simulink model "TestAccel"  (R2016a)
settings: Solver=FixedStepAuto  StartTime=0.0  StopTime=inf  FixedStep=1  RelTol=1e-3
libraries: arduinolib x1, EEE481Arduino x1
settings Model: ExtModeTrigDuration=2  Creator=rsjoshi1  LastModifiedBy=rsjoshi1
settings OptimizationCC: OptimizeModelRefInitCode=on  LifeSpan=1  MaxStackSize=64
settings HardwareCC: ProdBitPerPointer=32  ProdLargestAtomicInteger=Long  ProdLargestAtomicFloat=Double  ProdWordSize=32  ProdHWDeviceType=ARM Compatible->ARM Cortex
settings RTWCC: SystemTargetFile=ert.tlc  HardwareBoard=Arduino Due  TemplateMakefile=ert_default_tmf  GenerateReport=on  Toolchain=Arduino ARM v1.6.1  BuildConfiguration=Faster Runs  IncludeHyperlinkInReport=on  LaunchReport=on  GenerateTraceInfo=on  GenerateTraceReport=on  GenerateTraceReportSl=on  GenerateTraceReportSf=on  GenerateTraceReportEml=on
settings CodeAppCC: ForceParamTrailComments=on  IgnoreCustomStorageClasses=off  OperatorAnnotations=on  SimulinkDataObjDesc=on  SFDataObjDesc=on  MATLABFcnDesc=on  InsertBlockDesc=on  MATLABSourceComments=on
settings ERTTargetCC: SupportContinuousTime=on  SupportVariableSizeSignals=on

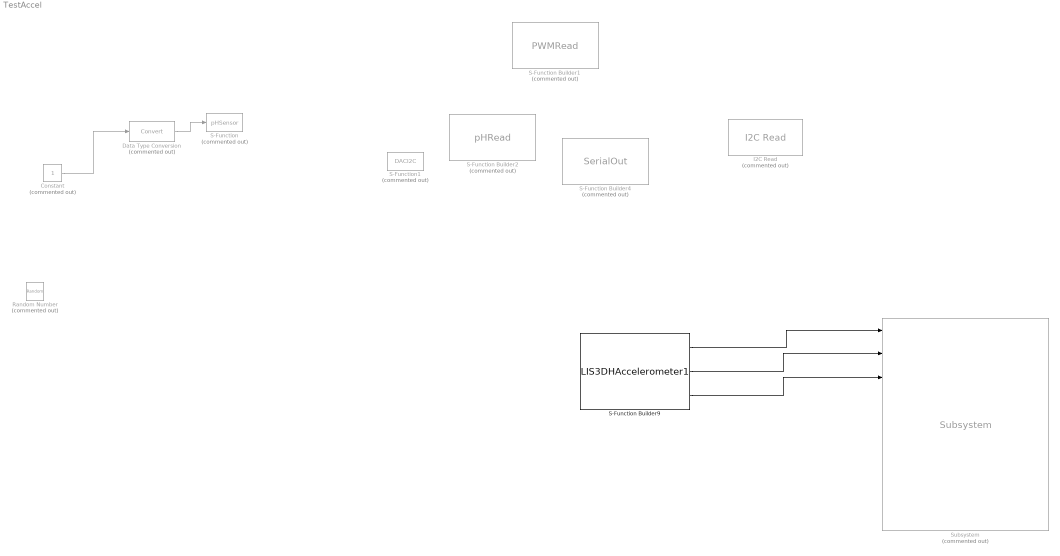
== system TestAccel ==
  Constant : Constant  Commented=on
  Data Type Conversion : DataTypeConversion  Commented=on
  I2C Read : arduinolib/I2C Read  Commented=on  SlaveAddress_=hex2dec( '61' )  RegisterAddressEnable=off  RegisterAddress_=hex2dec( '20' )  Datatype=uint8  ByteOrder=Big Endian  Datalength_=1  SampleTime_=1  blockPlatform=arduino
  Random Number : RandomNumber  Commented=on  SampleTime=0.1
  S-Function : S-Function  Commented=on  FunctionName=pHSensor  Parameters=int8(1)  SFunctionModules=pHSensor_wrapper  SFunctionDeploymentMode=off  EnableBusSupport=off
  S-Function Builder1 : S-Function  Commented=on  InitFcn=try, set_param(gcb,'FunctionName','PWMRead'), end  FunctionName=PWMRead  SFunctionModules=PWMRead_wrapper  SFunctionDeploymentMode=off  EnableBusSupport=off  mask(S-Function Builder){}
      mask help: Simulink:masks:SFunctionBuilder_MD
      mask init:
      | val = [[.9  0.75 0.75 1 1 .9 .9 1]',[1 1 0.75 0.75 .9 .9 1 .9]'];try , sys = get_param(gcb,'SfunBuilderFcnName');if isempty(sys), sys = get_param(gcb,'FunctionName'); end,catch, sys = get_param(gcb,'FunctionName'); end
      settings: CopyFcn=set_param(gcbh,'LinkStatus','none')  PreSaveFcn=try, set_param(gcb,'FunctionName','PWMRead'), end  OpenFcn=sfunctionwizard(gcbh)
      mask Display: plot(val(:,1),val(:,2)),disp(sys), port_label('output',1,'PWMValue')
  S-Function Builder2 : S-Function  Commented=on  InitFcn=try, set_param(gcb,'FunctionName','pHRead'), end  FunctionName=pHRead  Parameters=int8(1)  SFunctionModules=pHRead_wrapper  SFunctionDeploymentMode=off  EnableBusSupport=off  mask(S-Function Builder){}
      mask help: Simulink:masks:SFunctionBuilder_MD
      mask init: same as TestAccel/S-Function Builder1
      settings: CopyFcn=set_param(gcbh,'LinkStatus','none')  PreSaveFcn=try, set_param(gcb,'FunctionName','pHRead'), end  OpenFcn=sfunctionwizard(gcbh)
      mask Display: plot(val(:,1),val(:,2)),disp(sys), port_label('input',1,'CommandNumber'), port_label('input',2,'TriggerCommand'), port_label('output',1,'pHValue')
  S-Function Builder4 : S-Function  Commented=on  InitFcn=try, set_param(gcb,'FunctionName','SerialOut'), end  FunctionName=SerialOut  Parameters=int8(0)  SFunctionModules=SerialOut_wrapper  SFunctionDeploymentMode=off  EnableBusSupport=off  mask(S-Function Builder){}
      mask help: Simulink:masks:SFunctionBuilder_MD
      mask init: same as TestAccel/S-Function Builder1
      settings: CopyFcn=set_param(gcbh,'LinkStatus','none')  PreSaveFcn=try, set_param(gcb,'FunctionName','SerialOut'), end  OpenFcn=sfunctionwizard(gcbh)
      mask Display: plot(val(:,1),val(:,2)),disp(sys), port_label('input',1,'input')
  S-Function Builder9 : S-Function  InitFcn=try, set_param(gcb,'FunctionName','LIS3DHAccelerometer1'), end  FunctionName=LIS3DHAccelerometer1  Parameters=int8(1),int8(1)  SFunctionModules=LIS3DHAccelerometer1_wrapper  SFunctionDeploymentMode=off  EnableBusSupport=off  mask(S-Function Builder){}
      mask help: Simulink:masks:SFunctionBuilder_MD
      mask init: same as TestAccel/S-Function Builder1
      settings: CopyFcn=set_param(gcbh,'LinkStatus','none')  PreSaveFcn=try, set_param(gcb,'FunctionName','LIS3DHAccelerometer1'), end  OpenFcn=sfunctionwizard(gcbh)
      mask Display: plot(val(:,1),val(:,2)),disp(sys), port_label('output',1,'AccX'), port_label('output',2,'AccY'), port_label('output',3,'AccZ')
  S-Function1 : S-Function  Commented=on  FunctionName=DACI2C  SFunctionModules=DACI2C_wrapper  SFunctionDeploymentMode=off  EnableBusSupport=off
  Subsystem : EEE481Arduino/Subsystem  Commented=on  Tsa=1  rate=0
  wires:
  Constant/1 -> Data Type Conversion/1
  Data Type Conversion/1 -> S-Function/1
  S-Function Builder9/1 -> Subsystem/1
  S-Function Builder9/2 -> Subsystem/2
  S-Function Builder9/3 -> Subsystem/3
